simulink model "rle_sim_stickGMT"  (R2020b)
settings: Solver=FixedStepDiscrete  StartTime=0.0  StopTime=sssha_acc_dt.time(end)  FixedStep=FEM_Ts  MaxStep=FEM_Ts  RelTol=1e-2
InitFcn:
  | %
  | % Initialization callback function
  | %
  | 
  | try
  |    fprintf('\nGMT IMS version (%s)!\n',simulink_fname );
  | 
  |    % Get Simulink model directory
  |    [filepath,name,ext] = fileparts(which(bdroot));
  | 
  |    if ~strcmp(filepath,pwd)
  |       fprintf('\nChanging current directory to \n %s \n',filepath);
  |       cd(filepath);
  |    end
  | 
  |    %
  |  if(osim.bpless_wl)
  |     fprintf('Generating bumpless wind load time series\n');
  |  end
  | catch
  |    warning('Running the InitFcn from puSimulate script');
  | end
values from neighbouring files (symbols this model uses):
  FEM_Ts = 1/1e3    (= 0.001)    [load_rle_sim_stickGMT.m]
  PG = zeros(length(om2),6)    [load_rle_sim_stickGMT.m]
  phiB = inputs2ModalF(mode_ind_vec,indDesInputs)    [load_rle_sim_stickGMT.m]
  phiC = modalDisp2Outputs(indDesOutputs,mode_ind_vec)    [load_rle_sim_stickGMT.m]
  Psi_ss = gainMatrix(indDesOutputs,indDesInputs) - K_ss    [load_rle_sim_stickGMT.m]
settings Model: SimulationMode=accelerator  Creator=RRomano  LastModifiedBy=rromano
settings SolverCC: MaxConsecutiveMinStep=10  ZeroCrossAlgorithm=Adaptive
settings DataIOCC: SaveOutput=off  SignalLogging=off  DSMLogging=off  SaveTime=off  ReturnWorkspaceOutputs=off
settings OptimizationCC: DefaultParameterBehavior=Inlined  StrengthReduction=on  PassReuseOutputArgsAs=Individual arguments  EfficientMapNaN2IntZero=off  SimCompilerOptimization=on  AccelVerboseBuild=on  OptimizeBlockOrder=speed  OptimizationPriority=Speed  OptimizationCustomize=off  MultiThreadedLoops=on  EfficientTunableParamExpr=on
settings DebuggingCC: InheritedTsInSrcMsg=none  MultiTaskRateTransMsg=warning  ParameterTunabilityLossMsg=error  SFUnexpectedBacktrackingDiag=warning  SFNoUnconditionalDefaultTransitionDiag=warning  SFExecutionAtInitializationDiag=none  ArithmeticOperatorsInVariantConditions=warning
settings HardwareCC: ProdBitPerLong=64  ProdHWDeviceType=Intel->x86-64 (Linux 64)  TargetBitPerLong=64  TargetBitPerPointer=64  TargetBitPerSizeT=64  TargetBitPerPtrDiffT=64  TargetLongLongMode=on  TargetIntDivRoundTo=Zero  TargetEndianess=LittleEndian  TargetWordSize=64  TargetHWDeviceType=MATLAB Host  ProdEqTarget=off
settings SFSimCC: SimUseLocalCustomCode=off  MATLABDynamicMemAlloc=off  CustomCodeUndefinedFunction=UseInterfaceOnly
settings RTWCC: Description=Embedded Coder  SystemTargetFile=ert.tlc  GenCodeOnly=on  TemplateMakefile=ert_default_tmf  GenerateReport=on  BuildConfiguration=Faster Runs  IncludeHyperlinkInReport=on  GenerateTraceInfo=on  GenerateTraceReport=on  GenerateTraceReportSl=on  GenerateTraceReportSf=on  GenerateTraceReportEml=on
settings CodeAppCC: ForceParamTrailComments=on  IgnoreCustomStorageClasses=off  MaxIdLength=128  OperatorAnnotations=on  SimulinkDataObjDesc=on  SFDataObjDesc=on  InsertBlockDesc=on  MATLABSourceComments=on
settings ERTTargetCC: GenerateSampleERTMain=on  InlinedParameterPlacement=NonHierarchical  ERTCustomFileTemplate=example_file_process.tlc
settings ConfigComp: CovMetricSettings=dw  CovSaveCumulativeToWorkspaceVar=on  CovSaveSingleToWorkspaceVar=on  CovExternalEMLEnable=off

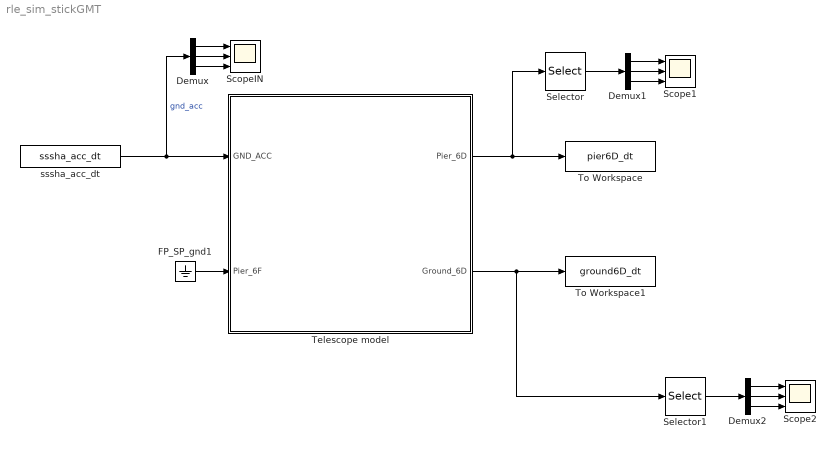
== system rle_sim_stickGMT ==
  Demux : Demux  Outputs=3
  Demux1 : Demux  Outputs=3
  Demux2 : Demux  Outputs=3
  FP_SP_gnd1 : Ground
  Scope1 : Scope  NumInputPorts=3
  Scope2 : Scope  NumInputPorts=3
  ScopeIN : Scope  NumInputPorts=3
  Selector : Selector  InputPortWidth=12  IndexOptions=Index vector (dialog)  Indices=[1:3]  OutputSizes=1
  Selector1 : Selector  InputPortWidth=6  IndexOptions=Index vector (dialog)  Indices=[1:3]  OutputSizes=1
  Telescope model : Subsystem
  To Workspace : ToWorkspace  VariableName=pier6D_dt  SampleTime=-1
  To Workspace1 : ToWorkspace  VariableName=ground6D_dt  SampleTime=-1
  sssha_acc_dt : FromWorkspace  VariableName=sssha_acc_dt  Interpolate=off  OutputAfterFinalValue=Setting to zero
  wires:
  FP_SP_gnd1/1 -> Telescope model/2(Pier_6F)
  Demux/3 -> ScopeIN/3
  Demux/2 -> ScopeIN/2
  Demux/1 -> ScopeIN/1
  sssha_acc_dt/1 -> Demux/1, Telescope model/1(GND_ACC)  "gnd_acc"
  Telescope model/1(Pier_6D) -> Selector/1, To Workspace/1
  Demux1/2 -> Scope1/2
  Demux1/1 -> Scope1/1
  Demux1/3 -> Scope1/3
  Selector/1 -> Demux1/1
  Demux2/1 -> Scope2/1
  Selector1/1 -> Demux2/1
  Demux2/2 -> Scope2/2
  Telescope model/2(Ground_6D) -> Selector1/1, To Workspace1/1
  Demux2/3 -> Scope2/3

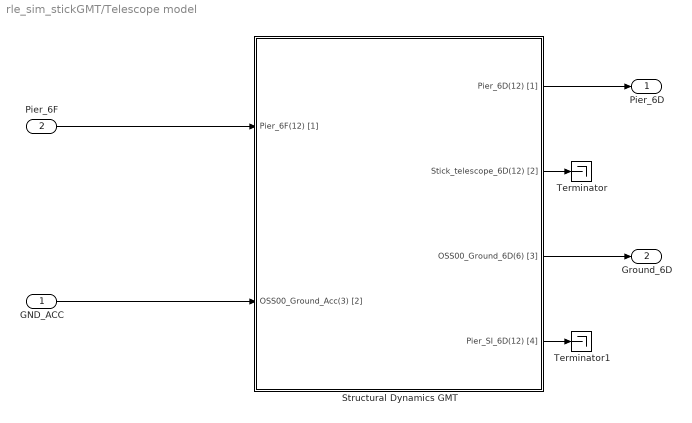
== system rle_sim_stickGMT/Telescope model ==
  GND_ACC : Inport
  Pier_6F : Inport  Port=2
  Structural Dynamics GMT : Subsystem
  Terminator : Terminator
  Terminator1 : Terminator
  Pier_6D : Outport  VectorParamsAs1DForOutWhenUnconnected=off
  Ground_6D : Outport  Port=2  VectorParamsAs1DForOutWhenUnconnected=off
  wires:
  GND_ACC/1 -> Structural Dynamics GMT/2(OSS00_Ground_Acc(3) [2])
  Pier_6F/1 -> Structural Dynamics GMT/1(Pier_6F(12) [1])
  Structural Dynamics GMT/1(Pier_6D(12) [1]) -> Pier_6D/1
  Structural Dynamics GMT/3(OSS00_Ground_6D(6) [3]) -> Ground_6D/1
  Structural Dynamics GMT/2(Stick_telescope_6D(12) [2]) -> Terminator/1
  Structural Dynamics GMT/4(Pier_SI_6D(12) [4]) -> Terminator1/1

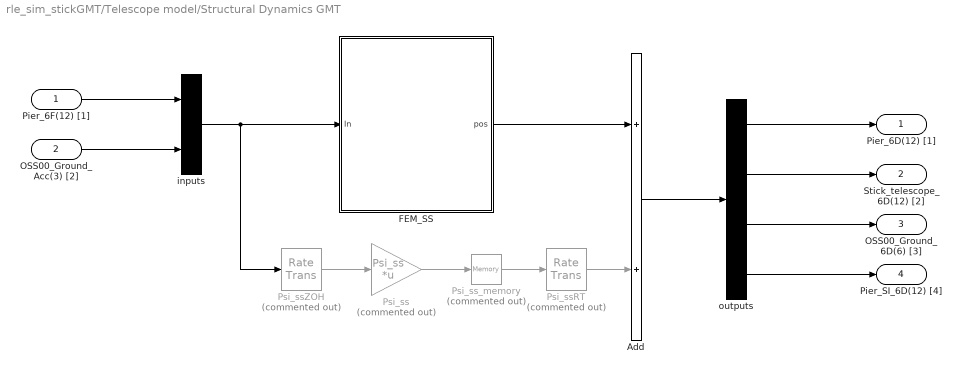
== system rle_sim_stickGMT/Telescope model/Structural Dynamics GMT ==
  Pier_6F(12) [1] : Inport  PortDimensions=12
  OSS00_Ground_Acc(3) [2] : Inport  Port=2  PortDimensions=3
  Add : Sum
  FEM_SS : Subsystem
  Psi_ss : Gain  Commented=on  Gain=Psi_ss  Multiplication=Matrix(K*u) (u vector)
  Psi_ssRT : RateTransition  Commented=on  Integrity=off  OutPortSampleTimeOpt=Inherit
  Psi_ssZOH : RateTransition  Commented=on  Integrity=off  OutPortSampleTime=Psi_ssTs
  Psi_ss_memory : Memory  Commented=on  InitialCondition=zeros(size(phiC,1),1)  InheritSampleTime=on  LinearizeAsDelay=on
  inputs : Mux  Inputs=modelMuxDims
  outputs : Demux  Outputs=modelDemuxDims
  Pier_6D(12) [1] : Outport  PortDimensions=12
  Stick_telescope_6D(12) [2] : Outport  Port=2  PortDimensions=12
  OSS00_Ground_6D(6) [3] : Outport  Port=3  PortDimensions=6
  Pier_SI_6D(12) [4] : Outport  Port=4  PortDimensions=12
  wires:
  outputs/4 -> Pier_SI_6D(12) [4]/1
  outputs/3 -> OSS00_Ground_6D(6) [3]/1
  outputs/2 -> Stick_telescope_6D(12) [2]/1
  outputs/1 -> Pier_6D(12) [1]/1
  Add/1 -> outputs/1
  OSS00_Ground_Acc(3) [2]/1 -> inputs/2
  Pier_6F(12) [1]/1 -> inputs/1
  Psi_ssZOH/1 -> Psi_ss/1
  FEM_SS/1(pos) -> Add/1
  Psi_ss_memory/1 -> Psi_ssRT/1
  inputs/1 -> Psi_ssZOH/1, FEM_SS/1(In)
  Psi_ss/1 -> Psi_ss_memory/1
  Psi_ssRT/1 -> Add/2

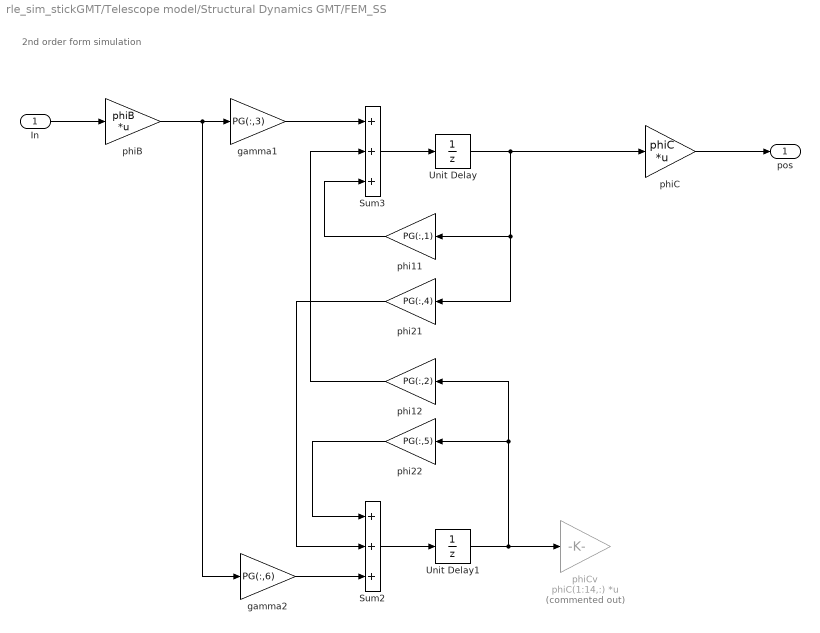
== system rle_sim_stickGMT/Telescope model/Structural Dynamics GMT/FEM_SS ==
  note: 2nd order form simulation
  In : Inport
  Sum2 : Sum  Inputs=+++
  Sum3 : Sum  Inputs=+++
  Unit Delay : UnitDelay  SampleTime=FEM_Ts  HasFrameUpgradeWarning=on
  Unit Delay1 : UnitDelay  SampleTime=FEM_Ts  HasFrameUpgradeWarning=on
  gamma1 : Gain  Gain=PG(:,3)
  gamma2 : Gain  Gain=PG(:,6)
  phi11 : Gain  Gain=PG(:,1)
  phi12 : Gain  Gain=PG(:,2)
  phi21 : Gain  Gain=PG(:,4)
  phi22 : Gain  Gain=PG(:,5)
  phiB : Gain  Gain=phiB  Multiplication=Matrix(K*u) (u vector)
  phiC : Gain  Gain=phiC  Multiplication=Matrix(K*u) (u vector)
  phiCv : Gain  Commented=on  Gain=phiC(1:14,:)  Multiplication=Matrix(K*u) (u vector)
  pos : Outport  VectorParamsAs1DForOutWhenUnconnected=off
  wires:
  Unit Delay/1 -> phi11/1, phi21/1, phiC/1
  phi12/1 -> Sum3/2
  Sum2/1 -> Unit Delay1/1
  Sum3/1 -> Unit Delay/1
  gamma2/1 -> Sum2/3
  phi21/1 -> Sum2/2
  phi22/1 -> Sum2/1
  gamma1/1 -> Sum3/1
  phi11/1 -> Sum3/3
  Unit Delay1/1 -> phiCv/1, phi12/1, phi22/1
  phiB/1 -> gamma2/1, gamma1/1
  phiC/1 -> pos/1
  In/1 -> phiB/1
